simulink model "HLSDem_SelectParameter"  (R2016b)
settings: configuration reference "CodeGenConfigSet" (kept outside this file)
values from neighbouring files (symbols this model uses):
  HLSDem_facFdbkLoGrip_C = Calibration.Parameter    [init_HLSDem_SelectParameter.m]    (also in init_HLSDem_SelectParameter_SIL.m = Simulink.Parameter)
  HLSDem_facFdbkLoNoGrip_C = Calibration.Parameter    [init_HLSDem_SelectParameter.m]    (also in init_HLSDem_SelectParameter_SIL.m = Simulink.Parameter)
  HLSDem_facFdbkTrqLosHiGrip_CUR = Calibration.Parameter    [init_HLSDem_SelectParameter.m]    (also in init_HLSDem_SelectParameter_SIL.m = Simulink.Parameter)
  HLSDem_facFdbkTrqLosHiGrip_CURX = Calibration.Parameter    [init_HLSDem_SelectParameter.m]    (also in init_HLSDem_SelectParameter_SIL.m = Simulink.Parameter)
  HLSDem_facFdbkTrqLosHiNoGrip_C = Calibration.Parameter    [init_HLSDem_SelectParameter.m]    (also in init_HLSDem_SelectParameter_SIL.m = Simulink.Parameter)
  HLSDem_facFdbkTrqLosLoGrip_CUR = Calibration.Parameter    [init_HLSDem_SelectParameter.m]    (also in init_HLSDem_SelectParameter_SIL.m = Simulink.Parameter)
  HLSDem_facFdbkTrqLosLoGrip_CURX = Calibration.Parameter    [init_HLSDem_SelectParameter.m]    (also in init_HLSDem_SelectParameter_SIL.m = Simulink.Parameter)
  HLSDem_facFdbkTrqLosLoNoGrip_C = Calibration.Parameter    [init_HLSDem_SelectParameter.m]    (also in init_HLSDem_SelectParameter_SIL.m = Simulink.Parameter)
  HLSDem_facNAvrgPT1_C = Calibration.Parameter    [init_HLSDem_SelectParameter.m]    (also in init_HLSDem_SelectParameter_SIL.m = Simulink.Parameter)
  HLSDem_facTrqPT1CorFac_C = Calibration.Parameter    [init_HLSDem_SelectParameter.m]    (also in init_HLSDem_SelectParameter_SIL.m = Simulink.Parameter)
  HLSDem_GripIKiHi_CUR = Calibration.Parameter    [init_HLSDem_SelectParameter.m]    (also in init_HLSDem_SelectParameter_SIL.m = Simulink.Parameter)
  HLSDem_GripIKiHi_CURX = Calibration.Parameter    [init_HLSDem_SelectParameter.m]    (also in init_HLSDem_SelectParameter_SIL.m = Simulink.Parameter)
  HLSDem_GripIKiLo_CUR = Calibration.Parameter    [init_HLSDem_SelectParameter.m]    (also in init_HLSDem_SelectParameter_SIL.m = Simulink.Parameter)
  HLSDem_GripIKiLo_CURX = Calibration.Parameter    [init_HLSDem_SelectParameter.m]    (also in init_HLSDem_SelectParameter_SIL.m = Simulink.Parameter)
  HLSDem_GripIKiNegHi_CUR = Calibration.Parameter    [init_HLSDem_SelectParameter.m]    (also in init_HLSDem_SelectParameter_SIL.m = Simulink.Parameter)
  HLSDem_GripIKiNegHi_CURX = Calibration.Parameter    [init_HLSDem_SelectParameter.m]    (also in init_HLSDem_SelectParameter_SIL.m = Simulink.Parameter)
  HLSDem_GripIKiNegLo_CUR = Calibration.Parameter    [init_HLSDem_SelectParameter.m]    (also in init_HLSDem_SelectParameter_SIL.m = Simulink.Parameter)
  HLSDem_GripIKiNegLo_CURX = Calibration.Parameter    [init_HLSDem_SelectParameter.m]    (also in init_HLSDem_SelectParameter_SIL.m = Simulink.Parameter)
  HLSDem_GripIKiPosHi_CUR = Calibration.Parameter    [init_HLSDem_SelectParameter.m]    (also in init_HLSDem_SelectParameter_SIL.m = Simulink.Parameter)
  HLSDem_GripIKiPosHi_CURX = Calibration.Parameter    [init_HLSDem_SelectParameter.m]    (also in init_HLSDem_SelectParameter_SIL.m = Simulink.Parameter)
  HLSDem_GripIKiPosLo_CUR = Calibration.Parameter    [init_HLSDem_SelectParameter.m]    (also in init_HLSDem_SelectParameter_SIL.m = Simulink.Parameter)
  HLSDem_GripIKiPosLo_CURX = Calibration.Parameter    [init_HLSDem_SelectParameter.m]    (also in init_HLSDem_SelectParameter_SIL.m = Simulink.Parameter)
  HLSDem_GripIWinNegHi_C = Calibration.Parameter    [init_HLSDem_SelectParameter.m]    (also in init_HLSDem_SelectParameter_SIL.m = Simulink.Parameter)
  HLSDem_GripIWinNegLo_C = Calibration.Parameter    [init_HLSDem_SelectParameter.m]    (also in init_HLSDem_SelectParameter_SIL.m = Simulink.Parameter)
  HLSDem_GripIWinPosHi_C = Calibration.Parameter    [init_HLSDem_SelectParameter.m]    (also in init_HLSDem_SelectParameter_SIL.m = Simulink.Parameter)
  HLSDem_GripIWinPosLo_C = Calibration.Parameter    [init_HLSDem_SelectParameter.m]    (also in init_HLSDem_SelectParameter_SIL.m = Simulink.Parameter)
  HLSDem_GripPKpHi_CUR = Calibration.Parameter    [init_HLSDem_SelectParameter.m]    (also in init_HLSDem_SelectParameter_SIL.m = Simulink.Parameter)
  HLSDem_GripPKpHi_CURX = Calibration.Parameter    [init_HLSDem_SelectParameter.m]    (also in init_HLSDem_SelectParameter_SIL.m = Simulink.Parameter)
  HLSDem_GripPKpLo_CUR = Calibration.Parameter    [init_HLSDem_SelectParameter.m]    (also in init_HLSDem_SelectParameter_SIL.m = Simulink.Parameter)
  HLSDem_GripPKpLo_CURX = Calibration.Parameter    [init_HLSDem_SelectParameter.m]    (also in init_HLSDem_SelectParameter_SIL.m = Simulink.Parameter)
  HLSDem_GripPKpNegHi_CUR = Calibration.Parameter    [init_HLSDem_SelectParameter.m]    (also in init_HLSDem_SelectParameter_SIL.m = Simulink.Parameter)
  HLSDem_GripPKpNegHi_CURX = Calibration.Parameter    [init_HLSDem_SelectParameter.m]    (also in init_HLSDem_SelectParameter_SIL.m = Simulink.Parameter)
  HLSDem_GripPKpNegLo_CUR = Calibration.Parameter    [init_HLSDem_SelectParameter.m]    (also in init_HLSDem_SelectParameter_SIL.m = Simulink.Parameter)
  HLSDem_GripPKpNegLo_CURX = Calibration.Parameter    [init_HLSDem_SelectParameter.m]    (also in init_HLSDem_SelectParameter_SIL.m = Simulink.Parameter)
  HLSDem_GripPKpPosHi_CUR = Calibration.Parameter    [init_HLSDem_SelectParameter.m]    (also in init_HLSDem_SelectParameter_SIL.m = Simulink.Parameter)
  HLSDem_GripPKpPosHi_CURX = Calibration.Parameter    [init_HLSDem_SelectParameter.m]    (also in init_HLSDem_SelectParameter_SIL.m = Simulink.Parameter)
  HLSDem_GripPKpPosLo_CUR = Calibration.Parameter    [init_HLSDem_SelectParameter.m]    (also in init_HLSDem_SelectParameter_SIL.m = Simulink.Parameter)
  HLSDem_GripPKpPosLo_CURX = Calibration.Parameter    [init_HLSDem_SelectParameter.m]    (also in init_HLSDem_SelectParameter_SIL.m = Simulink.Parameter)
  HLSDem_GripPWinNegHi_C = Calibration.Parameter    [init_HLSDem_SelectParameter.m]    (also in init_HLSDem_SelectParameter_SIL.m = Simulink.Parameter)
  HLSDem_GripPWinNegLo_C = Calibration.Parameter    [init_HLSDem_SelectParameter.m]    (also in init_HLSDem_SelectParameter_SIL.m = Simulink.Parameter)
  HLSDem_GripPWinPosHi_C = Calibration.Parameter    [init_HLSDem_SelectParameter.m]    (also in init_HLSDem_SelectParameter_SIL.m = Simulink.Parameter)
  HLSDem_GripPWinPosLo_C = Calibration.Parameter    [init_HLSDem_SelectParameter.m]    (also in init_HLSDem_SelectParameter_SIL.m = Simulink.Parameter)
  HLSDem_InrtVehGrip_CUR = Calibration.Parameter    [init_HLSDem_SelectParameter.m]    (also in init_HLSDem_SelectParameter_SIL.m = Simulink.Parameter)
  HLSDem_InrtVehGrip_CURX = Calibration.Parameter    [init_HLSDem_SelectParameter.m]    (also in init_HLSDem_SelectParameter_SIL.m = Simulink.Parameter)
  HLSDem_InrtVehNoGrip_C = Calibration.Parameter    [init_HLSDem_SelectParameter.m]    (also in init_HLSDem_SelectParameter_SIL.m = Simulink.Parameter)
  HLSDem_KiCorFac_MAP = Calibration.Parameter    [init_HLSDem_SelectParameter.m]    (also in init_HLSDem_SelectParameter_SIL.m = Simulink.Parameter)
  HLSDem_KiCorFac_MAPX = Calibration.Parameter    [init_HLSDem_SelectParameter.m]    (also in init_HLSDem_SelectParameter_SIL.m = Simulink.Parameter)
  HLSDem_KiCorFac_MAPY = Calibration.Parameter    [init_HLSDem_SelectParameter.m]    (also in init_HLSDem_SelectParameter_SIL.m = Simulink.Parameter)
  HLSDem_KiCorTrqFac_MAP = Calibration.Parameter    [init_HLSDem_SelectParameter.m]    (also in init_HLSDem_SelectParameter_SIL.m = Simulink.Parameter)
  HLSDem_KiCorTrqFac_MAPX = Calibration.Parameter    [init_HLSDem_SelectParameter.m]    (also in init_HLSDem_SelectParameter_SIL.m = Simulink.Parameter)
  HLSDem_KiCorTrqFac_MAPY = Calibration.Parameter    [init_HLSDem_SelectParameter.m]    (also in init_HLSDem_SelectParameter_SIL.m = Simulink.Parameter)
  HLSDem_KpCorFac_MAP = Calibration.Parameter    [init_HLSDem_SelectParameter.m]    (also in init_HLSDem_SelectParameter_SIL.m = Simulink.Parameter)
  HLSDem_KpCorFac_MAPX = Calibration.Parameter    [init_HLSDem_SelectParameter.m]    (also in init_HLSDem_SelectParameter_SIL.m = Simulink.Parameter)
  HLSDem_KpCorFac_MAPY = Calibration.Parameter    [init_HLSDem_SelectParameter.m]    (also in init_HLSDem_SelectParameter_SIL.m = Simulink.Parameter)
  HLSDem_KpCorTrqFac_MAP = Calibration.Parameter    [init_HLSDem_SelectParameter.m]    (also in init_HLSDem_SelectParameter_SIL.m = Simulink.Parameter)
  HLSDem_KpCorTrqFac_MAPX = Calibration.Parameter    [init_HLSDem_SelectParameter.m]    (also in init_HLSDem_SelectParameter_SIL.m = Simulink.Parameter)
  HLSDem_KpCorTrqFac_MAPY = Calibration.Parameter    [init_HLSDem_SelectParameter.m]    (also in init_HLSDem_SelectParameter_SIL.m = Simulink.Parameter)
  HLSDem_NoGripdnAccLim_C = Calibration.Parameter    [init_HLSDem_SelectParameter.m]    (also in init_HLSDem_SelectParameter_SIL.m = Simulink.Parameter)
  HLSDem_NoGripdnDeclLim_C = Calibration.Parameter    [init_HLSDem_SelectParameter.m]    (also in init_HLSDem_SelectParameter_SIL.m = Simulink.Parameter)
  HLSDem_NoGripdnDeclLimBrk_C = Calibration.Parameter    [init_HLSDem_SelectParameter.m]    (also in init_HLSDem_SelectParameter_SIL.m = Simulink.Parameter)
  HLSDem_NoGripIKiHi_C = Calibration.Parameter    [init_HLSDem_SelectParameter.m]    (also in init_HLSDem_SelectParameter_SIL.m = Simulink.Parameter)
  HLSDem_NoGripIKiLo_C = Calibration.Parameter    [init_HLSDem_SelectParameter.m]    (also in init_HLSDem_SelectParameter_SIL.m = Simulink.Parameter)
  HLSDem_NoGripIKiNegHi_C = Calibration.Parameter    [init_HLSDem_SelectParameter.m]    (also in init_HLSDem_SelectParameter_SIL.m = Simulink.Parameter)
  HLSDem_NoGripIKiNegLo_C = Calibration.Parameter    [init_HLSDem_SelectParameter.m]    (also in init_HLSDem_SelectParameter_SIL.m = Simulink.Parameter)
  HLSDem_NoGripIKiPosHi_C = Calibration.Parameter    [init_HLSDem_SelectParameter.m]    (also in init_HLSDem_SelectParameter_SIL.m = Simulink.Parameter)
  HLSDem_NoGripIKiPosLo_C = Calibration.Parameter    [init_HLSDem_SelectParameter.m]    (also in init_HLSDem_SelectParameter_SIL.m = Simulink.Parameter)
  HLSDem_NoGripIWinNegHi_C = Calibration.Parameter    [init_HLSDem_SelectParameter.m]    (also in init_HLSDem_SelectParameter_SIL.m = Simulink.Parameter)
  HLSDem_NoGripIWinNegLo_C = Calibration.Parameter    [init_HLSDem_SelectParameter.m]    (also in init_HLSDem_SelectParameter_SIL.m = Simulink.Parameter)
  HLSDem_NoGripIWinPosHi_C = Calibration.Parameter    [init_HLSDem_SelectParameter.m]    (also in init_HLSDem_SelectParameter_SIL.m = Simulink.Parameter)
  HLSDem_NoGripIWinPosLo_C = Calibration.Parameter    [init_HLSDem_SelectParameter.m]    (also in init_HLSDem_SelectParameter_SIL.m = Simulink.Parameter)
  HLSDem_NoGripPKpHi_C = Calibration.Parameter    [init_HLSDem_SelectParameter.m]    (also in init_HLSDem_SelectParameter_SIL.m = Simulink.Parameter)
  HLSDem_NoGripPKpLo_C = Calibration.Parameter    [init_HLSDem_SelectParameter.m]    (also in init_HLSDem_SelectParameter_SIL.m = Simulink.Parameter)
  HLSDem_NoGripPKpNegHi_C = Calibration.Parameter    [init_HLSDem_SelectParameter.m]    (also in init_HLSDem_SelectParameter_SIL.m = Simulink.Parameter)
  HLSDem_NoGripPKpNegLo_C = Calibration.Parameter    [init_HLSDem_SelectParameter.m]    (also in init_HLSDem_SelectParameter_SIL.m = Simulink.Parameter)
  HLSDem_NoGripPKpPosHi_C = Calibration.Parameter    [init_HLSDem_SelectParameter.m]    (also in init_HLSDem_SelectParameter_SIL.m = Simulink.Parameter)
  HLSDem_NoGripPKpPosLo_C = Calibration.Parameter    [init_HLSDem_SelectParameter.m]    (also in init_HLSDem_SelectParameter_SIL.m = Simulink.Parameter)
  HLSDem_NoGripPWinNegHi_C = Calibration.Parameter    [init_HLSDem_SelectParameter.m]    (also in init_HLSDem_SelectParameter_SIL.m = Simulink.Parameter)
  HLSDem_NoGripPWinNegLo_C = Calibration.Parameter    [init_HLSDem_SelectParameter.m]    (also in init_HLSDem_SelectParameter_SIL.m = Simulink.Parameter)
  HLSDem_NoGripPWinPosHi_C = Calibration.Parameter    [init_HLSDem_SelectParameter.m]    (also in init_HLSDem_SelectParameter_SIL.m = Simulink.Parameter)
  HLSDem_NoGripPWinPosLo_C = Calibration.Parameter    [init_HLSDem_SelectParameter.m]    (also in init_HLSDem_SelectParameter_SIL.m = Simulink.Parameter)
  HLSDem_rNoGripThres_C = Calibration.Parameter    [init_HLSDem_SelectParameter.m]    (also in init_HLSDem_SelectParameter_SIL.m = Simulink.Parameter)
  HLSDem_stBrkTrq_C = Calibration.Parameter    [init_HLSDem_SelectParameter.m]    (also in init_HLSDem_SelectParameter_SIL.m = Simulink.Parameter)
  HLSDem_swtTempSelParAdap_C = Calibration.Parameter    [init_HLSDem_SelectParameter.m]    (also in init_HLSDem_SelectParameter_SIL.m = Simulink.Parameter)
  HLSDem_swtTrqSelCorFac_C = Calibration.Parameter    [init_HLSDem_SelectParameter.m]    (also in init_HLSDem_SelectParameter_SIL.m = Simulink.Parameter)
  HLSDem_tiFltTrqLosGrip_CUR = Calibration.Parameter    [init_HLSDem_SelectParameter.m]    (also in init_HLSDem_SelectParameter_SIL.m = Simulink.Parameter)
  HLSDem_tiFltTrqLosGrip_CURX = Calibration.Parameter    [init_HLSDem_SelectParameter.m]    (also in init_HLSDem_SelectParameter_SIL.m = Simulink.Parameter)
  HLSDem_tiFltTrqLosNoGrip_C = Calibration.Parameter    [init_HLSDem_SelectParameter.m]    (also in init_HLSDem_SelectParameter_SIL.m = Simulink.Parameter)
libraries: CXLib x2
(part 1 of 2)
settings Model: Creator=Administrator  LastModifiedBy=xuxingpei
settings ConfigSetRef: SourceLocation=Base Workspace

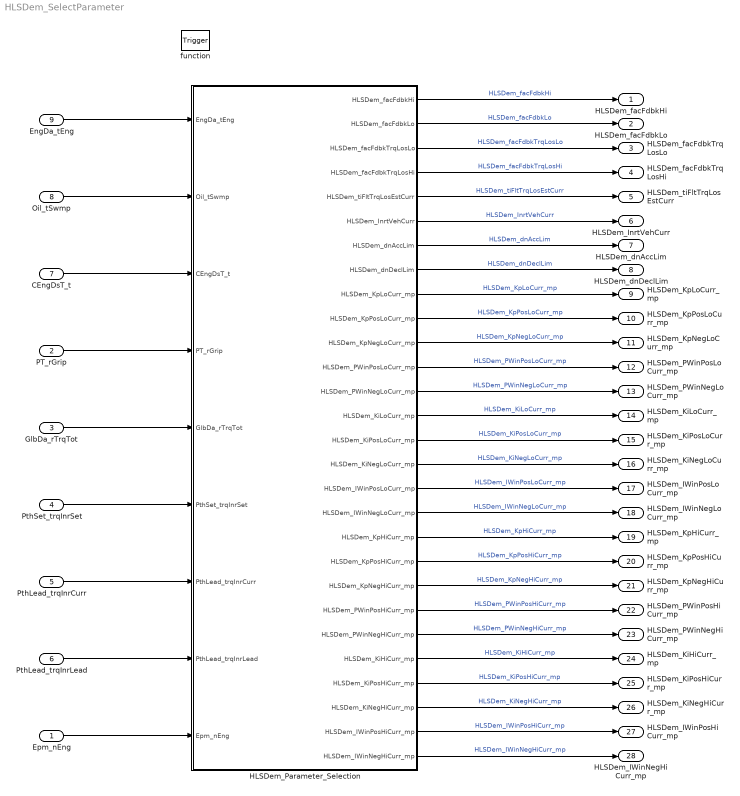
== system HLSDem_SelectParameter ==
  Epm_nEng : Inport  Tag=rpm  Description=Engine speed  OutMin=0  OutMax=6000  OutDataTypeStr=EngSpeed_rpm
  PT_rGrip : Inport  Description=Analogue value for the grip states  Port=2  OutMin=-300  OutMax=300  OutDataTypeStr=Prc_Fact100
  GlbDa_rTrqTot : Inport  Description=total ratio of the power train inclusive the differential and the converter torque ratio  Port=3  OutMin=-327  OutMax=327  OutDataTypeStr=TransRatio
  PthSet_trqInrSet : Inport  Tag=Nm  Description=Inner torque set value after monitoring limitation  Port=4  OutMin=-3000  OutMax=3276.7  OutDataTypeStr=Trq_Nm
  PthLead_trqInrCurr : Inport  Tag=Nm  Description=Actual percent engine torque  Port=5  OutMin=-3000  OutMax=3000  OutDataTypeStr=Trq_Nm
  PthLead_trqInrLead : Inport  Tag=Nm  Description=Inner torque lead value  Port=6  OutMin=-3000  OutMax=3000  OutDataTypeStr=Trq_Nm
  CEngDsT_t : Inport  Tag=deg  Description=engine coolant temperature after filter  Port=7  OutMin=-200  OutMax=200  OutDataTypeStr=Temp_deg
  Oil_tSwmp : Inport  Tag=deg  Description=Oil temperature in oil sump  Port=8  OutMin=-50  OutMax=200  OutDataTypeStr=Temp_deg
  EngDa_tEng : Inport  Tag=deg  Description=Engine temperature  Port=9  OutMin=-1000  OutMax=1000  OutDataTypeStr=Temp_deg
  function : TriggerPort  TriggerType=function-call  VariantControl=Variant
  HLSDem_Parameter_Selection : Subsystem
  HLSDem_facFdbkHi : Outport  Tag=rpm/Nm  Description=Feedback factor for the upper setpoint  OutMin=-20  OutMax=20  OutDataTypeStr=FdbkNm2rpm_rpm_Nm
  HLSDem_facFdbkLo : Outport  Tag=rpm/Nm  Description=Feedback factor for the lower setpoint  Port=2  OutMin=-20  OutMax=20  OutDataTypeStr=FdbkNm2rpm_rpm_Nm
  HLSDem_facFdbkTrqLosLo : Outport  Tag=rpm/Nm  Description=Inner feedback factor for the lower setpoint  Port=3  OutMin=-20  OutMax=20  OutDataTypeStr=FdbkNm2rpm_rpm_Nm
  HLSDem_facFdbkTrqLosHi : Outport  Tag=rpm/Nm  Description=Inner feedback factor for the upper setpoint  Port=4  OutMin=-20  OutMax=20  OutDataTypeStr=FdbkNm2rpm_rpm_Nm
  HLSDem_tiFltTrqLosEstCurr : Outport  Description=Time constant (PT1filter) for EISGov torque loss estimation  Port=5  OutMin=0  OutMax=99.998  OutDataTypeStr=PT_fac
  HLSDem_InrtVehCurr : Outport  Tag=Nm/(rpm/s)  Description=Mass Inertia for EISGov torque loss estimation  Port=6  OutMin=-50  OutMax=50  OutDataTypeStr=HLSDem_Inrt
  HLSDem_dnAccLim : Outport  Tag=rpm/s  Description=Maximum permissible acceleration (Engine speed)  Port=7  OutMin=-12000  OutMax=12000  OutDataTypeStr=EngSpeed_rpm_s
  HLSDem_dnDeclLim : Outport  Tag=rpm/s  Description=Maximum permissible deceleration (Engine speed)  Port=8  OutMin=-12000  OutMax=12000  OutDataTypeStr=EngSpeed_rpm_s
  HLSDem_KpLoCurr_mp : Outport  Tag=Nm/rpm  Description=Current gain of the P-element of lower path  Port=9  OutMin=-10000  OutMax=10000  OutDataTypeStr=HLSDem_Kp
  HLSDem_KpPosLoCurr_mp : Outport  Tag=Nm/rpm  Description=Current positive large signal gain of the P-element of lower path  Port=10  OutMin=-10000  OutMax=10000  OutDataTypeStr=HLSDem_Kp
  HLSDem_KpNegLoCurr_mp : Outport  Tag=Nm/rpm  Description=Current negative large signal gain of the P-element of lower path  Port=11  OutMin=-10000  OutMax=10000  OutDataTypeStr=HLSDem_Kp
  HLSDem_PWinPosLoCurr_mp : Outport  Tag=rpm  Description=Current positive small-signal window P-component of the lower path  Port=12  OutMin=-6000  OutMax=6000  OutDataTypeStr=EngSpeed_rpm
  HLSDem_PWinNegLoCurr_mp : Outport  Tag=rpm  Description=Current negative small-signal window P-component of the lower path  Port=13  OutMin=-6000  OutMax=6000  OutDataTypeStr=EngSpeed_rpm
  HLSDem_KiLoCurr_mp : Outport  Tag=Nm/(rpm*s)  Description=Current gain of the I-element of lower path  Port=14  OutMin=-18000  OutMax=18000  OutDataTypeStr=HLSDem_Ki
  HLSDem_KiPosLoCurr_mp : Outport  Tag=Nm/(rpm*s)  Description=Current positive large signal gain of the I-element of lower path  Port=15  OutMin=-18000  OutMax=18000  OutDataTypeStr=HLSDem_Ki
  HLSDem_KiNegLoCurr_mp : Outport  Tag=Nm/(rpm*s)  Description=Current negative large signal gain of the I-element of lower path  Port=16  OutMin=-18000  OutMax=18000  OutDataTypeStr=HLSDem_Ki
  HLSDem_IWinPosLoCurr_mp : Outport  Tag=rpm  Description=Current positive small-signal window I-component of the lower path  Port=17  OutMin=-6000  OutMax=6000  OutDataTypeStr=EngSpeed_rpm
  HLSDem_IWinNegLoCurr_mp : Outport  Tag=rpm  Description=Current negative small-signal window I-component of the lower path  Port=18  OutMin=-6000  OutMax=6000  OutDataTypeStr=EngSpeed_rpm
  HLSDem_KpHiCurr_mp : Outport  Tag=Nm/rpm  Description=Current gain of the P-element of upper path  Port=19  OutMin=-10000  OutMax=10000  OutDataTypeStr=HLSDem_Kp
  HLSDem_KpPosHiCurr_mp : Outport  Tag=Nm/rpm  Description=Current positive large signal gain of the P-element of upper path  Port=20  OutMin=-10000  OutMax=10000  OutDataTypeStr=HLSDem_Kp
  HLSDem_KpNegHiCurr_mp : Outport  Tag=Nm/rpm  Description=Current negative large signal gain of the P-element of upper path  Port=21  OutMin=-10000  OutMax=10000  OutDataTypeStr=HLSDem_Kp
  HLSDem_PWinPosHiCurr_mp : Outport  Tag=rpm  Description=Current positive small-signal window P-component of the upper path  Port=22  OutMin=-6000  OutMax=6000  OutDataTypeStr=EngSpeed_rpm
  HLSDem_PWinNegHiCurr_mp : Outport  Tag=rpm  Description=Current negative small-signal window P-component of the upper path  Port=23  OutMin=-6000  OutMax=6000  OutDataTypeStr=EngSpeed_rpm
  HLSDem_KiHiCurr_mp : Outport  Tag=Nm/(rpm*s)  Description=Current small signal gain for the I component upper PI - path  Port=24  OutMin=-18000  OutMax=18000  OutDataTypeStr=HLSDem_Ki
  HLSDem_KiPosHiCurr_mp : Outport  Tag=Nm/(rpm*s)  Description=Current positive large signal gain for the I component upper PI-path  Port=25  OutMin=-18000  OutMax=18000  OutDataTypeStr=HLSDem_Ki
  HLSDem_KiNegHiCurr_mp : Outport  Tag=Nm/(rpm*s)  Description=Current negative large signal gain for the I component upper PI - path  Port=26  OutMin=-18000  OutMax=18000  OutDataTypeStr=HLSDem_Ki
  HLSDem_IWinPosHiCurr_mp : Outport  Tag=rpm  Description=Current positive small-signal window I-component of the upper path  Port=27  OutMin=-6000  OutMax=6000  OutDataTypeStr=EngSpeed_rpm
  HLSDem_IWinNegHiCurr_mp : Outport  Tag=rpm  Description=Current negative small-signal window I-component of the upper path  Port=28  OutMin=-6000  OutMax=6000  OutDataTypeStr=EngSpeed_rpm
  wires:
  PT_rGrip/1 -> HLSDem_Parameter_Selection/4(PT_rGrip)
  PthSet_trqInrSet/1 -> HLSDem_Parameter_Selection/6(PthSet_trqInrSet)
  Epm_nEng/1 -> HLSDem_Parameter_Selection/9(Epm_nEng)
  PthLead_trqInrCurr/1 -> HLSDem_Parameter_Selection/7(PthLead_trqInrCurr)
  PthLead_trqInrLead/1 -> HLSDem_Parameter_Selection/8(PthLead_trqInrLead)
  GlbDa_rTrqTot/1 -> HLSDem_Parameter_Selection/5(GlbDa_rTrqTot)
  HLSDem_Parameter_Selection/1(HLSDem_facFdbkHi) -> HLSDem_facFdbkHi/1  "HLSDem_facFdbkHi"
  HLSDem_Parameter_Selection/2(HLSDem_facFdbkLo) -> HLSDem_facFdbkLo/1  "HLSDem_facFdbkLo"
  HLSDem_Parameter_Selection/3(HLSDem_facFdbkTrqLosLo) -> HLSDem_facFdbkTrqLosLo/1  "HLSDem_facFdbkTrqLosLo"
  HLSDem_Parameter_Selection/4(HLSDem_facFdbkTrqLosHi) -> HLSDem_facFdbkTrqLosHi/1  "HLSDem_facFdbkTrqLosHi"
  HLSDem_Parameter_Selection/5(HLSDem_tiFltTrqLosEstCurr) -> HLSDem_tiFltTrqLosEstCurr/1  "HLSDem_tiFltTrqLosEstCurr"
  HLSDem_Parameter_Selection/6(HLSDem_InrtVehCurr) -> HLSDem_InrtVehCurr/1  "HLSDem_InrtVehCurr"
  HLSDem_Parameter_Selection/7(HLSDem_dnAccLim) -> HLSDem_dnAccLim/1  "HLSDem_dnAccLim"
  HLSDem_Parameter_Selection/8(HLSDem_dnDeclLim) -> HLSDem_dnDeclLim/1  "HLSDem_dnDeclLim"
  HLSDem_Parameter_Selection/9(HLSDem_KpLoCurr_mp) -> HLSDem_KpLoCurr_mp/1  "HLSDem_KpLoCurr_mp"
  HLSDem_Parameter_Selection/10(HLSDem_KpPosLoCurr_mp) -> HLSDem_KpPosLoCurr_mp/1  "HLSDem_KpPosLoCurr_mp"
  HLSDem_Parameter_Selection/11(HLSDem_KpNegLoCurr_mp) -> HLSDem_KpNegLoCurr_mp/1  "HLSDem_KpNegLoCurr_mp"
  HLSDem_Parameter_Selection/12(HLSDem_PWinPosLoCurr_mp) -> HLSDem_PWinPosLoCurr_mp/1  "HLSDem_PWinPosLoCurr_mp"
  HLSDem_Parameter_Selection/13(HLSDem_PWinNegLoCurr_mp) -> HLSDem_PWinNegLoCurr_mp/1  "HLSDem_PWinNegLoCurr_mp"
  HLSDem_Parameter_Selection/14(HLSDem_KiLoCurr_mp) -> HLSDem_KiLoCurr_mp/1  "HLSDem_KiLoCurr_mp"
  HLSDem_Parameter_Selection/15(HLSDem_KiPosLoCurr_mp) -> HLSDem_KiPosLoCurr_mp/1  "HLSDem_KiPosLoCurr_mp"
  HLSDem_Parameter_Selection/16(HLSDem_KiNegLoCurr_mp) -> HLSDem_KiNegLoCurr_mp/1  "HLSDem_KiNegLoCurr_mp"
  HLSDem_Parameter_Selection/17(HLSDem_IWinPosLoCurr_mp) -> HLSDem_IWinPosLoCurr_mp/1  "HLSDem_IWinPosLoCurr_mp"
  HLSDem_Parameter_Selection/18(HLSDem_IWinNegLoCurr_mp) -> HLSDem_IWinNegLoCurr_mp/1  "HLSDem_IWinNegLoCurr_mp"
  HLSDem_Parameter_Selection/19(HLSDem_KpHiCurr_mp) -> HLSDem_KpHiCurr_mp/1  "HLSDem_KpHiCurr_mp"
  HLSDem_Parameter_Selection/20(HLSDem_KpPosHiCurr_mp) -> HLSDem_KpPosHiCurr_mp/1  "HLSDem_KpPosHiCurr_mp"
  HLSDem_Parameter_Selection/21(HLSDem_KpNegHiCurr_mp) -> HLSDem_KpNegHiCurr_mp/1  "HLSDem_KpNegHiCurr_mp"
  HLSDem_Parameter_Selection/22(HLSDem_PWinPosHiCurr_mp) -> HLSDem_PWinPosHiCurr_mp/1  "HLSDem_PWinPosHiCurr_mp"
  HLSDem_Parameter_Selection/23(HLSDem_PWinNegHiCurr_mp) -> HLSDem_PWinNegHiCurr_mp/1  "HLSDem_PWinNegHiCurr_mp"
  HLSDem_Parameter_Selection/24(HLSDem_KiHiCurr_mp) -> HLSDem_KiHiCurr_mp/1  "HLSDem_KiHiCurr_mp"
  HLSDem_Parameter_Selection/25(HLSDem_KiPosHiCurr_mp) -> HLSDem_KiPosHiCurr_mp/1  "HLSDem_KiPosHiCurr_mp"
  HLSDem_Parameter_Selection/26(HLSDem_KiNegHiCurr_mp) -> HLSDem_KiNegHiCurr_mp/1  "HLSDem_KiNegHiCurr_mp"
  HLSDem_Parameter_Selection/27(HLSDem_IWinPosHiCurr_mp) -> HLSDem_IWinPosHiCurr_mp/1  "HLSDem_IWinPosHiCurr_mp"
  HLSDem_Parameter_Selection/28(HLSDem_IWinNegHiCurr_mp) -> HLSDem_IWinNegHiCurr_mp/1  "HLSDem_IWinNegHiCurr_mp"
  CEngDsT_t/1 -> HLSDem_Parameter_Selection/3(CEngDsT_t)
  Oil_tSwmp/1 -> HLSDem_Parameter_Selection/2(Oil_tSwmp)
  EngDa_tEng/1 -> HLSDem_Parameter_Selection/1(EngDa_tEng)

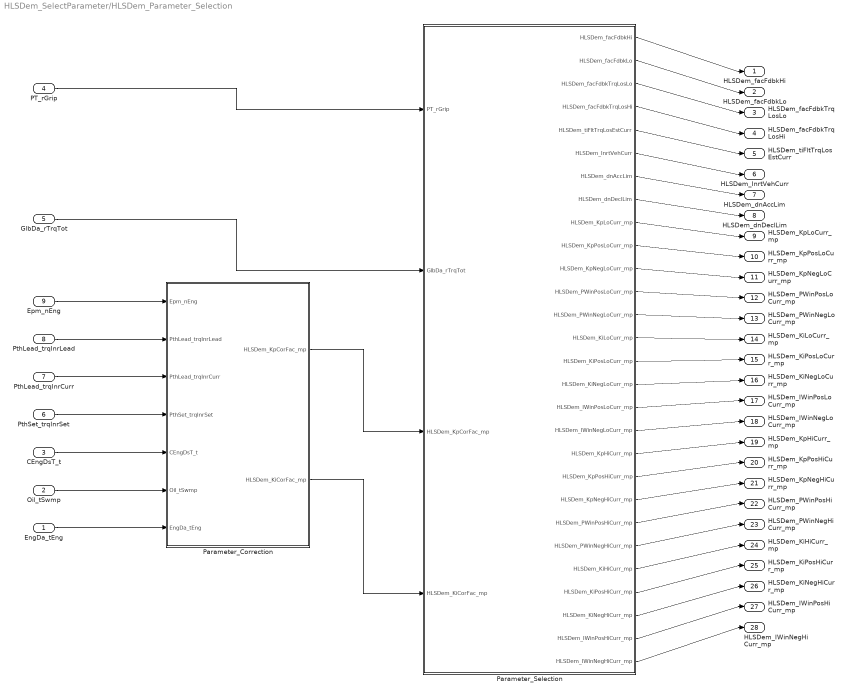
== system HLSDem_SelectParameter/HLSDem_Parameter_Selection ==
  EngDa_tEng : Inport  Tag=deg  Description=Engine temperature  OutMin=-1000  OutMax=1000  OutDataTypeStr=Temp_deg
  Oil_tSwmp : Inport  Tag=deg  Description=Oil temperature in oil sump  Port=2  OutMin=-50  OutMax=200  OutDataTypeStr=Temp_deg
  CEngDsT_t : Inport  Tag=deg  Description=engine coolant temperature after filter  Port=3  OutMin=-200  OutMax=200  OutDataTypeStr=Temp_deg
  PT_rGrip : Inport  Port=4
  GlbDa_rTrqTot : Inport  Port=5
  PthSet_trqInrSet : Inport  Port=6
  PthLead_trqInrCurr : Inport  Port=7
  PthLead_trqInrLead : Inport  Port=8
  Epm_nEng : Inport  Port=9
  Parameter_Correction : Subsystem
  Parameter_Selection : Subsystem
  HLSDem_facFdbkHi : Outport
  HLSDem_facFdbkLo : Outport  Port=2
  HLSDem_facFdbkTrqLosLo : Outport  Port=3
  HLSDem_facFdbkTrqLosHi : Outport  Port=4
  HLSDem_tiFltTrqLosEstCurr : Outport  Port=5
  HLSDem_InrtVehCurr : Outport  Port=6
  HLSDem_dnAccLim : Outport  Port=7
  HLSDem_dnDeclLim : Outport  Port=8
  HLSDem_KpLoCurr_mp : Outport  Port=9
  HLSDem_KpPosLoCurr_mp : Outport  Port=10
  HLSDem_KpNegLoCurr_mp : Outport  Port=11
  HLSDem_PWinPosLoCurr_mp : Outport  Port=12
  HLSDem_PWinNegLoCurr_mp : Outport  Port=13
  HLSDem_KiLoCurr_mp : Outport  Port=14
  HLSDem_KiPosLoCurr_mp : Outport  Port=15
  HLSDem_KiNegLoCurr_mp : Outport  Port=16
  HLSDem_IWinPosLoCurr_mp : Outport  Port=17
  HLSDem_IWinNegLoCurr_mp : Outport  Port=18
  HLSDem_KpHiCurr_mp : Outport  Port=19
  HLSDem_KpPosHiCurr_mp : Outport  Port=20
  HLSDem_KpNegHiCurr_mp : Outport  Port=21
  HLSDem_PWinPosHiCurr_mp : Outport  Port=22
  HLSDem_PWinNegHiCurr_mp : Outport  Port=23
  HLSDem_KiHiCurr_mp : Outport  Port=24
  HLSDem_KiPosHiCurr_mp : Outport  Port=25
  HLSDem_KiNegHiCurr_mp : Outport  Port=26
  HLSDem_IWinPosHiCurr_mp : Outport  Port=27
  HLSDem_IWinNegHiCurr_mp : Outport  Port=28
  wires:
  Parameter_Correction/2(HLSDem_KiCorFac_mp) -> Parameter_Selection/4(HLSDem_KiCorFac_mp)
  Epm_nEng/1 -> Parameter_Correction/1(Epm_nEng)
  PT_rGrip/1 -> Parameter_Selection/1(PT_rGrip)
  GlbDa_rTrqTot/1 -> Parameter_Selection/2(GlbDa_rTrqTot)
  PthLead_trqInrLead/1 -> Parameter_Correction/2(PthLead_trqInrLead)
  PthSet_trqInrSet/1 -> Parameter_Correction/4(PthSet_trqInrSet)
  PthLead_trqInrCurr/1 -> Parameter_Correction/3(PthLead_trqInrCurr)
  Parameter_Correction/1(HLSDem_KpCorFac_mp) -> Parameter_Selection/3(HLSDem_KpCorFac_mp)
  Parameter_Selection/1(HLSDem_facFdbkHi) -> HLSDem_facFdbkHi/1
  Parameter_Selection/2(HLSDem_facFdbkLo) -> HLSDem_facFdbkLo/1
  Parameter_Selection/3(HLSDem_facFdbkTrqLosLo) -> HLSDem_facFdbkTrqLosLo/1
  Parameter_Selection/4(HLSDem_facFdbkTrqLosHi) -> HLSDem_facFdbkTrqLosHi/1
  Parameter_Selection/5(HLSDem_tiFltTrqLosEstCurr) -> HLSDem_tiFltTrqLosEstCurr/1
  Parameter_Selection/6(HLSDem_InrtVehCurr) -> HLSDem_InrtVehCurr/1
  Parameter_Selection/7(HLSDem_dnAccLim) -> HLSDem_dnAccLim/1
  Parameter_Selection/8(HLSDem_dnDeclLim) -> HLSDem_dnDeclLim/1
  Parameter_Selection/9(HLSDem_KpLoCurr_mp) -> HLSDem_KpLoCurr_mp/1
  Parameter_Selection/10(HLSDem_KpPosLoCurr_mp) -> HLSDem_KpPosLoCurr_mp/1
  Parameter_Selection/11(HLSDem_KpNegLoCurr_mp) -> HLSDem_KpNegLoCurr_mp/1
  Parameter_Selection/12(HLSDem_PWinPosLoCurr_mp) -> HLSDem_PWinPosLoCurr_mp/1
  Parameter_Selection/13(HLSDem_PWinNegLoCurr_mp) -> HLSDem_PWinNegLoCurr_mp/1
  Parameter_Selection/14(HLSDem_KiLoCurr_mp) -> HLSDem_KiLoCurr_mp/1
  Parameter_Selection/15(HLSDem_KiPosLoCurr_mp) -> HLSDem_KiPosLoCurr_mp/1
  Parameter_Selection/16(HLSDem_KiNegLoCurr_mp) -> HLSDem_KiNegLoCurr_mp/1
  Parameter_Selection/17(HLSDem_IWinPosLoCurr_mp) -> HLSDem_IWinPosLoCurr_mp/1
  Parameter_Selection/18(HLSDem_IWinNegLoCurr_mp) -> HLSDem_IWinNegLoCurr_mp/1
  Parameter_Selection/19(HLSDem_KpHiCurr_mp) -> HLSDem_KpHiCurr_mp/1
  Parameter_Selection/20(HLSDem_KpPosHiCurr_mp) -> HLSDem_KpPosHiCurr_mp/1
  Parameter_Selection/21(HLSDem_KpNegHiCurr_mp) -> HLSDem_KpNegHiCurr_mp/1
  Parameter_Selection/22(HLSDem_PWinPosHiCurr_mp) -> HLSDem_PWinPosHiCurr_mp/1
  Parameter_Selection/23(HLSDem_PWinNegHiCurr_mp) -> HLSDem_PWinNegHiCurr_mp/1
  Parameter_Selection/24(HLSDem_KiHiCurr_mp) -> HLSDem_KiHiCurr_mp/1
  Parameter_Selection/25(HLSDem_KiPosHiCurr_mp) -> HLSDem_KiPosHiCurr_mp/1
  Parameter_Selection/26(HLSDem_KiNegHiCurr_mp) -> HLSDem_KiNegHiCurr_mp/1
  Parameter_Selection/27(HLSDem_IWinPosHiCurr_mp) -> HLSDem_IWinPosHiCurr_mp/1
  Parameter_Selection/28(HLSDem_IWinNegHiCurr_mp) -> HLSDem_IWinNegHiCurr_mp/1
  Oil_tSwmp/1 -> Parameter_Correction/6(Oil_tSwmp)
  EngDa_tEng/1 -> Parameter_Correction/7(EngDa_tEng)
  CEngDsT_t/1 -> Parameter_Correction/5(CEngDsT_t)

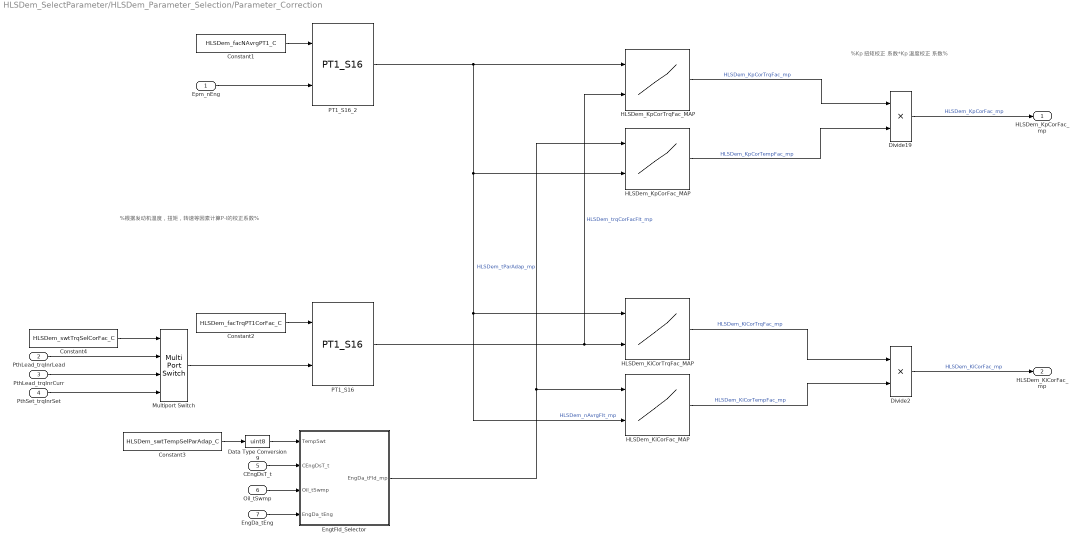
== system HLSDem_SelectParameter/HLSDem_Parameter_Selection/Parameter_Correction ==
  note: %Kp 扭矩校正 系数*Kp 温度校正 系数%
  note: %根据发动机温度，扭矩，转速等因素计算P-I的校正系数%
  Epm_nEng : Inport
  PthLead_trqInrLead : Inport  Port=2
  PthLead_trqInrCurr : Inport  Port=3
  PthSet_trqInrSet : Inport  Port=4
  CEngDsT_t : Inport  Tag=deg  Description=engine coolant temperature after filter  Port=5  OutMin=-200  OutMax=200  OutDataTypeStr=Temp_deg
  Oil_tSwmp : Inport  Tag=deg  Description=Oil temperature in oil sump  Port=6  OutMin=-50  OutMax=200  OutDataTypeStr=Temp_deg
  EngDa_tEng : Inport  Tag=deg  Description=Engine temperature  Port=7  OutMin=-1000  OutMax=1000  OutDataTypeStr=Temp_deg
  Constant1 : Constant  Value=HLSDem_facNAvrgPT1_C
  Constant2 : Constant  Value=HLSDem_facTrqPT1CorFac_C
  Constant3 : Constant  Value=HLSDem_swtTempSelParAdap_C
  Constant4 : Constant  Value=HLSDem_swtTrqSelCorFac_C
  Data Type Conversion9 : DataTypeConversion  OutDataTypeStr=uint8
  Divide19 : Product  Inputs=**  OutDataTypeStr=Factor  SaturateOnIntegerOverflow=on
  Divide2 : Product  Inputs=**  OutDataTypeStr=Factor  SaturateOnIntegerOverflow=on
  EngtFld_Selector : Subsystem
  HLSDem_KiCorFac_MAP : Lookup_n-D  BreakpointsForDimension1=HLSDem_KiCorFac_MAPY  BreakpointsForDimension2=HLSDem_KiCorFac_MAPX  Table=HLSDem_KiCorFac_MAP  ExtrapMethod=Clip  InternalRulePriority=Speed  OutDataTypeStr=Inherit: Inherit via back propagation  RndMeth=Simplest  SaturateOnIntegerOverflow=on
  HLSDem_KiCorTrqFac_MAP : Lookup_n-D  BreakpointsForDimension1=HLSDem_KiCorTrqFac_MAPY  BreakpointsForDimension2=HLSDem_KiCorTrqFac_MAPX  Table=HLSDem_KiCorTrqFac_MAP  ExtrapMethod=Clip  InternalRulePriority=Speed  OutDataTypeStr=Inherit: Inherit via back propagation  RndMeth=Simplest  SaturateOnIntegerOverflow=on
  HLSDem_KpCorFac_MAP : Lookup_n-D  BreakpointsForDimension1=HLSDem_KpCorFac_MAPY  BreakpointsForDimension2=HLSDem_KpCorFac_MAPX  Table=HLSDem_KpCorFac_MAP  ExtrapMethod=Clip  InternalRulePriority=Speed  OutDataTypeStr=Inherit: Inherit via back propagation  RndMeth=Simplest  SaturateOnIntegerOverflow=on
  HLSDem_KpCorTrqFac_MAP : Lookup_n-D  BreakpointsForDimension1=HLSDem_KpCorTrqFac_MAPY  BreakpointsForDimension2=HLSDem_KpCorTrqFac_MAPX  Table=HLSDem_KpCorTrqFac_MAP  ExtrapMethod=Clip  InternalRulePriority=Speed  OutDataTypeStr=Inherit: Inherit via back propagation  RndMeth=Simplest  SaturateOnIntegerOverflow=on
  Multiport Switch : MultiPortSwitch  DataPortOrder=Specify indices  DataPortIndices={2,1,0}
  PT1_S16 : CXLib/PT1_S16
  PT1_S16_2 : CXLib/PT1_S16
  HLSDem_KpCorFac_mp : Outport
  HLSDem_KiCorFac_mp : Outport  Port=2
  wires:
  PT1_S16/1 -> HLSDem_KiCorTrqFac_MAP/2, HLSDem_KpCorTrqFac_MAP/2  "HLSDem_trqCorFacFlt_mp"
  PthLead_trqInrCurr/1 -> Multiport Switch/3
  Epm_nEng/1 -> PT1_S16_2/2
  HLSDem_KiCorTrqFac_MAP/1 -> Divide2/1  "HLSDem_KiCorTrqFac_mp"
  Multiport Switch/1 -> PT1_S16/2
  PthSet_trqInrSet/1 -> Multiport Switch/4
  Constant4/1 -> Multiport Switch/1
  Constant1/1 -> PT1_S16_2/1
  HLSDem_KpCorFac_MAP/1 -> Divide19/2  "HLSDem_KpCorTempFac_mp"
  HLSDem_KiCorFac_MAP/1 -> Divide2/2  "HLSDem_KiCorTempFac_mp"
  Divide19/1 -> HLSDem_KpCorFac_mp/1  "HLSDem_KpCorFac_mp"
  Constant3/1 -> Data Type Conversion9/1
  HLSDem_KpCorTrqFac_MAP/1 -> Divide19/1  "HLSDem_KpCorTrqFac_mp"
  EngtFld_Selector/1(EngDa_tFld_mp) -> HLSDem_KiCorFac_MAP/1, HLSDem_KpCorFac_MAP/1  "HLSDem_tParAdap_mp"
  PT1_S16_2/1 -> HLSDem_KiCorFac_MAP/2, HLSDem_KiCorTrqFac_MAP/1, HLSDem_KpCorFac_MAP/2, HLSDem_KpCorTrqFac_MAP/1  "HLSDem_nAvrgFlt_mp"
  PthLead_trqInrLead/1 -> Multiport Switch/2
  Constant2/1 -> PT1_S16/1
  Divide2/1 -> HLSDem_KiCorFac_mp/1  "HLSDem_KiCorFac_mp"
  Data Type Conversion9/1 -> EngtFld_Selector/1(TempSwt)
  CEngDsT_t/1 -> EngtFld_Selector/2(CEngDsT_t)
  Oil_tSwmp/1 -> EngtFld_Selector/3(Oil_tSwmp)
  EngDa_tEng/1 -> EngtFld_Selector/4(EngDa_tEng)

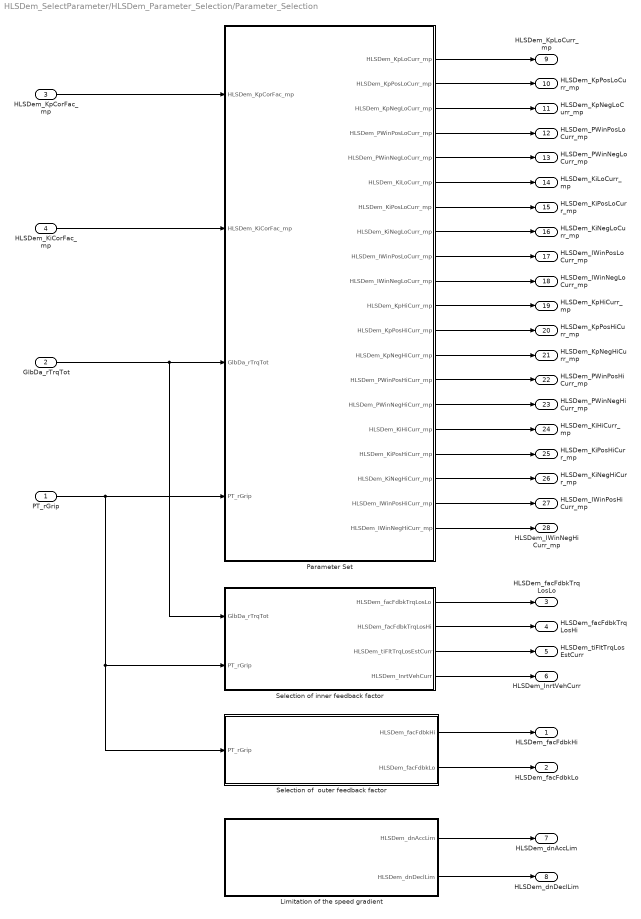
== system HLSDem_SelectParameter/HLSDem_Parameter_Selection/Parameter_Selection ==
  PT_rGrip : Inport
  GlbDa_rTrqTot : Inport  Port=2
  HLSDem_KpCorFac_mp : Inport  Port=3
  HLSDem_KiCorFac_mp : Inport  Port=4
  Limitation of the speed gradient : Subsystem
  Parameter Set : Subsystem
  Selection of  outer feedback factor : Subsystem
  Selection of inner feedback factor : Subsystem
  HLSDem_facFdbkHi : Outport
  HLSDem_facFdbkLo : Outport  Port=2
  HLSDem_facFdbkTrqLosLo : Outport  Port=3
  HLSDem_facFdbkTrqLosHi : Outport  Port=4
  HLSDem_tiFltTrqLosEstCurr : Outport  Port=5
  HLSDem_InrtVehCurr : Outport  Port=6
  HLSDem_dnAccLim : Outport  Port=7
  HLSDem_dnDeclLim : Outport  Port=8
  HLSDem_KpLoCurr_mp : Outport  Port=9
  HLSDem_KpPosLoCurr_mp : Outport  Port=10
  HLSDem_KpNegLoCurr_mp : Outport  Port=11
  HLSDem_PWinPosLoCurr_mp : Outport  Port=12
  HLSDem_PWinNegLoCurr_mp : Outport  Port=13
  HLSDem_KiLoCurr_mp : Outport  Port=14
  HLSDem_KiPosLoCurr_mp : Outport  Port=15
  HLSDem_KiNegLoCurr_mp : Outport  Port=16
  HLSDem_IWinPosLoCurr_mp : Outport  Port=17
  HLSDem_IWinNegLoCurr_mp : Outport  Port=18
  HLSDem_KpHiCurr_mp : Outport  Port=19
  HLSDem_KpPosHiCurr_mp : Outport  Port=20
  HLSDem_KpNegHiCurr_mp : Outport  Port=21
  HLSDem_PWinPosHiCurr_mp : Outport  Port=22
  HLSDem_PWinNegHiCurr_mp : Outport  Port=23
  HLSDem_KiHiCurr_mp : Outport  Port=24
  HLSDem_KiPosHiCurr_mp : Outport  Port=25
  HLSDem_KiNegHiCurr_mp : Outport  Port=26
  HLSDem_IWinPosHiCurr_mp : Outport  Port=27
  HLSDem_IWinNegHiCurr_mp : Outport  Port=28
  wires:
  Limitation of the speed gradient/2(HLSDem_dnDeclLim) -> HLSDem_dnDeclLim/1
  HLSDem_KiCorFac_mp/1 -> Parameter Set/2(HLSDem_KiCorFac_mp)
  Selection of  outer feedback factor/2(HLSDem_facFdbkLo) -> HLSDem_facFdbkLo/1
  Limitation of the speed gradient/1(HLSDem_dnAccLim) -> HLSDem_dnAccLim/1
  Selection of  outer feedback factor/1(HLSDem_facFdbkHi) -> HLSDem_facFdbkHi/1
  Selection of inner feedback factor/4(HLSDem_InrtVehCurr) -> HLSDem_InrtVehCurr/1
  Selection of inner feedback factor/3(HLSDem_tiFltTrqLosEstCurr) -> HLSDem_tiFltTrqLosEstCurr/1
  Selection of inner feedback factor/2(HLSDem_facFdbkTrqLosHi) -> HLSDem_facFdbkTrqLosHi/1
  PT_rGrip/1 -> Selection of  outer feedback factor/1(PT_rGrip), Selection of inner feedback factor/2(PT_rGrip), Parameter Set/4(PT_rGrip)
  Selection of inner feedback factor/1(HLSDem_facFdbkTrqLosLo) -> HLSDem_facFdbkTrqLosLo/1
  GlbDa_rTrqTot/1 -> Parameter Set/3(GlbDa_rTrqTot), Selection of inner feedback factor/1(GlbDa_rTrqTot)
  HLSDem_KpCorFac_mp/1 -> Parameter Set/1(HLSDem_KpCorFac_mp)
  Parameter Set/13(HLSDem_KpNegHiCurr_mp) -> HLSDem_KpNegHiCurr_mp/1
  Parameter Set/2(HLSDem_KpPosLoCurr_mp) -> HLSDem_KpPosLoCurr_mp/1
  Parameter Set/7(HLSDem_KiPosLoCurr_mp) -> HLSDem_KiPosLoCurr_mp/1
  Parameter Set/20(HLSDem_IWinNegHiCurr_mp) -> HLSDem_IWinNegHiCurr_mp/1
  Parameter Set/15(HLSDem_PWinNegHiCurr_mp) -> HLSDem_PWinNegHiCurr_mp/1
  Parameter Set/11(HLSDem_KpHiCurr_mp) -> HLSDem_KpHiCurr_mp/1
  Parameter Set/4(HLSDem_PWinPosLoCurr_mp) -> HLSDem_PWinPosLoCurr_mp/1
  Parameter Set/6(HLSDem_KiLoCurr_mp) -> HLSDem_KiLoCurr_mp/1
  Parameter Set/3(HLSDem_KpNegLoCurr_mp) -> HLSDem_KpNegLoCurr_mp/1
  Parameter Set/8(HLSDem_KiNegLoCurr_mp) -> HLSDem_KiNegLoCurr_mp/1
  Parameter Set/5(HLSDem_PWinNegLoCurr_mp) -> HLSDem_PWinNegLoCurr_mp/1
  Parameter Set/9(HLSDem_IWinPosLoCurr_mp) -> HLSDem_IWinPosLoCurr_mp/1
  Parameter Set/17(HLSDem_KiPosHiCurr_mp) -> HLSDem_KiPosHiCurr_mp/1
  Parameter Set/19(HLSDem_IWinPosHiCurr_mp) -> HLSDem_IWinPosHiCurr_mp/1
  Parameter Set/10(HLSDem_IWinNegLoCurr_mp) -> HLSDem_IWinNegLoCurr_mp/1
  Parameter Set/1(HLSDem_KpLoCurr_mp) -> HLSDem_KpLoCurr_mp/1
  Parameter Set/12(HLSDem_KpPosHiCurr_mp) -> HLSDem_KpPosHiCurr_mp/1
  Parameter Set/14(HLSDem_PWinPosHiCurr_mp) -> HLSDem_PWinPosHiCurr_mp/1
  Parameter Set/16(HLSDem_KiHiCurr_mp) -> HLSDem_KiHiCurr_mp/1
  Parameter Set/18(HLSDem_KiNegHiCurr_mp) -> HLSDem_KiNegHiCurr_mp/1

== system HLSDem_SelectParameter/HLSDem_Parameter_Selection/Parameter_Correction/EngtFld_Selector ==
  TempSwt : Inport
  CEngDsT_t : Inport  Tag=deg  Description=engine coolant temperature after filter  Port=2
  Oil_tSwmp : Inport  Tag=deg  Description=Oil temperature in oil sump  Port=3
  EngDa_tEng : Inport  Tag=deg  Description=Engine temperature  Port=4
  Data Type Conversion : DataTypeConversion  OutDataTypeStr=uint8
  Multiport Switch : MultiPortSwitch  DataPortOrder=Zero-based contiguous
  EngDa_tFld_mp : Outport  Tag=deg  Description=Engine temperature field
  wires:
  CEngDsT_t/1 -> Multiport Switch/2
  Multiport Switch/1 -> EngDa_tFld_mp/1
  EngDa_tEng/1 -> Multiport Switch/4
  Oil_tSwmp/1 -> Multiport Switch/3
  Data Type Conversion/1 -> Multiport Switch/1
  TempSwt/1 -> Data Type Conversion/1

== system HLSDem_SelectParameter/HLSDem_Parameter_Selection/Parameter_Selection/Limitation of the speed gradient ==
  note: %configured=0%
  note: %减速梯度限值%
  note: %加速梯度限值%
  note: %正常情况下减速%
  note: %踩刹车减速%
  Constant1 : Constant  Value=HLSDem_NoGripdnAccLim_C
  Constant2 : Constant  Value=HLSDem_NoGripdnDeclLimBrk_C
  Constant4 : Constant  Value=0  OutDataTypeStr=Inherit: Inherit via back propagation
  Constant5 : Constant  Value=HLSDem_NoGripdnDeclLim_C
  Constant6 : Constant  Value=HLSDem_stBrkTrq_C
  Relational Operator1 : RelationalOperator  Operator=>  OutDataTypeStr=boolean  RndMeth=Nearest  InputSameDT=on
  Signal Conversion : SignalConversion  OverrideOpt=off
  Switch3 : Switch  Criteria=u2 ~= 0  InputSameDT=on
  HLSDem_dnAccLim : Outport
  HLSDem_dnDeclLim : Outport  Port=2
  wires:
  Constant4/1 -> Relational Operator1/2
  Constant6/1 -> Relational Operator1/1
  Constant2/1 -> Switch3/1
  Relational Operator1/1 -> Switch3/2
  Constant5/1 -> Switch3/3
  Switch3/1 -> HLSDem_dnDeclLim/1
  Constant1/1 -> Signal Conversion/1
  Signal Conversion/1 -> HLSDem_dnAccLim/1

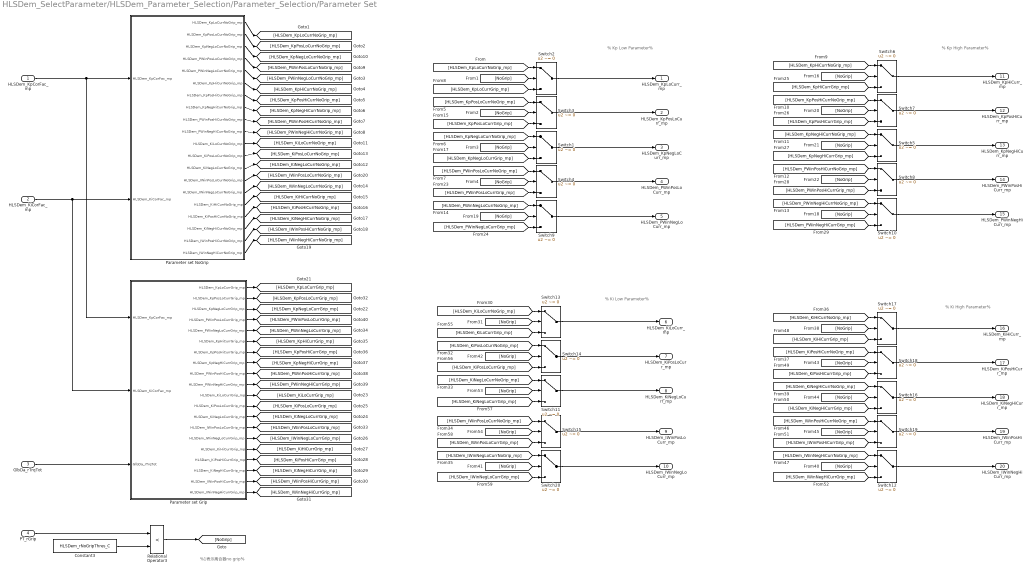
== system HLSDem_SelectParameter/HLSDem_Parameter_Selection/Parameter_Selection/Parameter Set ==
  note: %1表示离合器no grip%
  note: % Ki High Parameter%
  note: % Ki Low Parameter%
  note: % Kp High Parameter%
  note: % Kp Low Parameter%
  HLSDem_KpCorFac_mp : Inport
  HLSDem_KiCorFac_mp : Inport  Port=2
  GlbDa_rTrqTot : Inport  Port=3
  PT_rGrip : Inport  Port=4
  Constant3 : Constant  Value=HLSDem_rNoGripThres_C
  Parameter set Grip : Subsystem
  "Parameter set NoGrip " : Subsystem
  Relational Operator3 : RelationalOperator  Operator=<  OutDataTypeStr=boolean  RndMeth=Nearest
  Switch{1,3..20} (19 alike) : Switch  Criteria=u2 ~= 0
  Switch2 : Switch  Criteria=u2 ~= 0  InputSameDT=on
  HLSDem_KpLoCurr_mp : Outport
  HLSDem_KpPosLoCurr_mp : Outport  Port=2
  HLSDem_KpNegLoCurr_mp : Outport  Port=3
  HLSDem_PWinPosLoCurr_mp : Outport  Port=4
  HLSDem_PWinNegLoCurr_mp : Outport  Port=5
  HLSDem_KiLoCurr_mp : Outport  Port=6
  HLSDem_KiPosLoCurr_mp : Outport  Port=7
  HLSDem_KiNegLoCurr_mp : Outport  Port=8
  HLSDem_IWinPosLoCurr_mp : Outport  Port=9
  HLSDem_IWinNegLoCurr_mp : Outport  Port=10
  HLSDem_KpHiCurr_mp : Outport  Port=11
  HLSDem_KpPosHiCurr_mp : Outport  Port=12
  HLSDem_KpNegHiCurr_mp : Outport  Port=13
  HLSDem_PWinPosHiCurr_mp : Outport  Port=14
  HLSDem_PWinNegHiCurr_mp : Outport  Port=15
  HLSDem_KiHiCurr_mp : Outport  Port=16
  HLSDem_KiPosHiCurr_mp : Outport  Port=17
  HLSDem_KiNegHiCurr_mp : Outport  Port=18
  HLSDem_IWinPosHiCurr_mp : Outport  Port=19
  HLSDem_IWinNegHiCurr_mp : Outport  Port=20
  wires:
  Parameter set Grip/5(HLSDem_PWinNegLoCurrGrip_mp) -> [HLSDem_PWinNegLoCurrGrip_mp]
  Constant3/1 -> Relational Operator3/2
  "Parameter set NoGrip "/3(HLSDem_KpNegLoCurrNoGrip_mp) -> [HLSDem_KpNegLoCurrNoGrip_mp]
  Parameter set Grip/12(HLSDem_KiPosLoCurrGrip_mp) -> [HLSDem_KiPosLoCurrGrip_mp]
  "Parameter set NoGrip "/10(HLSDem_PWinNegHiCurrNoGrip_mp) -> [HLSDem_PWinNegHiCurrNoGrip_mp]
  Parameter set Grip/3(HLSDem_KpNegLoCurrGrip_mp) -> [HLSDem_KpNegLoCurrGrip_mp]
  Parameter set Grip/7(HLSDem_KpPosHiCurrGrip_mp) -> [HLSDem_KpPosHiCurrGrip_mp]
  "Parameter set NoGrip "/12(HLSDem_KiPosLoCurrNoGrip_mp) -> [HLSDem_KiPosLoCurrNoGrip_mp]
  "Parameter set NoGrip "/16(HLSDem_KiHiCurrNoGrip_mp) -> [HLSDem_KiHiCurrNoGrip_mp]
  "Parameter set NoGrip "/14(HLSDem_IWinPosLoCurrNoGrip_mp) -> [HLSDem_IWinPosLoCurrNoGrip_mp]
  Parameter set Grip/15(HLSDem_IWinNegLoCurrGrip_mp) -> [HLSDem_IWinNegLoCurrGrip_mp]
  Parameter set Grip/19(HLSDem_IWinPosHiCurrGrip_mp) -> [HLSDem_IWinPosHiCurrGrip_mp]
  "Parameter set NoGrip "/2(HLSDem_KpPosLoCurrNoGrip_mp) -> [HLSDem_KpPosLoCurrNoGrip_mp]
  HLSDem_KiCorFac_mp/1 -> Parameter set Grip/2(HLSDem_KiCorFac_mp), "Parameter set NoGrip "/2(HLSDem_KiCorFac_mp)
  Parameter set Grip/11(HLSDem_KiLoCurrGrip_mp) -> [HLSDem_KiLoCurrGrip_mp]
  Parameter set Grip/6(HLSDem_KpHiCurrGrip_mp) -> [HLSDem_KpHiCurrGrip_mp]
  "Parameter set NoGrip "/8(HLSDem_KpNegHiCurrNoGrip_mp) -> [HLSDem_KpNegHiCurrNoGrip_mp]
  HLSDem_KpCorFac_mp/1 -> Parameter set Grip/1(HLSDem_KpCorFac_mp), "Parameter set NoGrip "/1(HLSDem_KpCorFac_mp)
  Parameter set Grip/20(HLSDem_IWinNegHiCurrGrip_mp) -> [HLSDem_IWinNegHiCurrGrip_mp]
  "Parameter set NoGrip "/13(HLSDem_KiNegLoCurrNoGrip_mp) -> [HLSDem_KiNegLoCurrNoGrip_mp]
  Relational Operator3/1 -> [NoGrip]
  PT_rGrip/1 -> Relational Operator3/1
  Parameter set Grip/17(HLSDem_KiPosHiCurrGrip_mp) -> [HLSDem_KiPosHiCurrGrip_mp]
  Parameter set Grip/18(HLSDem_KiNegHiCurrGrip_mp) -> [HLSDem_KiNegHiCurrGrip_mp]
  GlbDa_rTrqTot/1 -> Parameter set Grip/3(GlbDa_rTrqTot)
  "Parameter set NoGrip "/15(HLSDem_IWinNegLoCurrNoGrip_mp) -> [HLSDem_IWinNegLoCurrNoGrip_mp]
  "Parameter set NoGrip "/19(HLSDem_IWinPosHiCurrNoGrip_mp) -> [HLSDem_IWinPosHiCurrNoGrip_mp]
  "Parameter set NoGrip "/20(HLSDem_IWinNegHiCurrNoGrip_mp) -> [HLSDem_IWinNegHiCurrNoGrip_mp]
  "Parameter set NoGrip "/1(HLSDem_KpLoCurrNoGrip_mp) -> [HLSDem_KpLoCurrNoGrip_mp]
  Parameter set Grip/1(HLSDem_KpLoCurrGrip_mp) -> [HLSDem_KpLoCurrGrip_mp]
  Parameter set Grip/14(HLSDem_IWinPosLoCurrGrip_mp) -> [HLSDem_IWinPosLoCurrGrip_mp]
  Parameter set Grip/16(HLSDem_KiHiCurrGrip_mp) -> [HLSDem_KiHiCurrGrip_mp]
  Parameter set Grip/9(HLSDem_PWinPosHiCurrGrip_mp) -> [HLSDem_PWinPosHiCurrGrip_mp]
  Parameter set Grip/13(HLSDem_KiNegLoCurrGrip_mp) -> [HLSDem_KiNegLoCurrGrip_mp]
  "Parameter set NoGrip "/4(HLSDem_PWinPosLoCurrNoGrip_mp) -> [HLSDem_PWinPosLoCurrNoGrip_mp]
  Parameter set Grip/4(HLSDem_PWinPosLoCurrGrip_mp) -> [HLSDem_PWinPosLoCurrGrip_mp]
  Parameter set Grip/2(HLSDem_KpPosLoCurrGrip_mp) -> [HLSDem_KpPosLoCurrGrip_mp]
  "Parameter set NoGrip "/17(HLSDem_KiPosHiCurrNoGrip_mp) -> [HLSDem_KiPosHiCurrNoGrip_mp]
  "Parameter set NoGrip "/6(HLSDem_KpHiCurrNoGrip_mp) -> [HLSDem_KpHiCurrNoGrip_mp]
  Parameter set Grip/10(HLSDem_PWinNegHiCurrGrip_mp) -> [HLSDem_PWinNegHiCurrGrip_mp]
  "Parameter set NoGrip "/5(HLSDem_PWinNegLoCurrNoGrip_mp) -> [HLSDem_PWinNegLoCurrNoGrip_mp]
  Parameter set Grip/8(HLSDem_KpNegHiCurrGrip_mp) -> [HLSDem_KpNegHiCurrGrip_mp]
  "Parameter set NoGrip "/7(HLSDem_KpPosHiCurrNoGrip_mp) -> [HLSDem_KpPosHiCurrNoGrip_mp]
  "Parameter set NoGrip "/18(HLSDem_KiNegHiCurrNoGrip_mp) -> [HLSDem_KiNegHiCurrNoGrip_mp]
  "Parameter set NoGrip "/11(HLSDem_KiLoCurrNoGrip_mp) -> [HLSDem_KiLoCurrNoGrip_mp]
  "Parameter set NoGrip "/9(HLSDem_PWinPosHiCurrNoGrip_mp) -> [HLSDem_PWinPosHiCurrNoGrip_mp]
  Switch18/1 -> HLSDem_KiPosHiCurr_mp/1
  Switch16/1 -> HLSDem_KiNegHiCurr_mp/1
  [NoGrip] -> Switch19/2
  Switch17/1 -> HLSDem_KiHiCurr_mp/1
  [NoGrip] -> Switch16/2
  [NoGrip] -> Switch12/2
  [HLSDem_KpLoCurrNoGrip_mp] -> Switch2/1
  Switch12/1 -> HLSDem_IWinNegHiCurr_mp/1
  [HLSDem_KiHiCurrNoGrip_mp] -> Switch17/1
  [HLSDem_KiNegLoCurrGrip_mp] -> Switch11/3
  [HLSDem_KiPosHiCurrNoGrip_mp] -> Switch18/1
  [HLSDem_IWinPosHiCurrNoGrip_mp] -> Switch19/1
  [HLSDem_KiNegHiCurrNoGrip_mp] -> Switch16/1
  [HLSDem_KiPosLoCurrGrip_mp] -> Switch14/3
  [HLSDem_KiLoCurrGrip_mp] -> Switch13/3
  Switch19/1 -> HLSDem_IWinPosHiCurr_mp/1
  [NoGrip] -> Switch18/2
  [HLSDem_IWinPosHiCurrGrip_mp] -> Switch19/3
  [HLSDem_IWinNegHiCurrGrip_mp] -> Switch12/3
  [HLSDem_KiPosHiCurrGrip_mp] -> Switch18/3
  [HLSDem_KiNegHiCurrGrip_mp] -> Switch16/3
  [HLSDem_KiHiCurrGrip_mp] -> Switch17/3
  [HLSDem_KiPosLoCurrNoGrip_mp] -> Switch14/1
  [HLSDem_IWinNegHiCurrNoGrip_mp] -> Switch12/1
  [HLSDem_KiLoCurrNoGrip_mp] -> Switch13/1
  [HLSDem_IWinPosLoCurrNoGrip_mp] -> Switch15/1
  [HLSDem_PWinNegLoCurrGrip_mp] -> Switch9/3
  [HLSDem_KpHiCurrGrip_mp] -> Switch6/3
  [HLSDem_KpPosLoCurrGrip_mp] -> Switch3/3
  [HLSDem_KpNegLoCurrGrip_mp] -> Switch1/3
  [HLSDem_PWinPosLoCurrGrip_mp] -> Switch4/3
  [HLSDem_KpPosHiCurrGrip_mp] -> Switch7/3
  [HLSDem_KpNegHiCurrNoGrip_mp] -> Switch5/1
  [NoGrip] -> Switch15/2
  [HLSDem_PWinNegHiCurrGrip_mp] -> Switch10/3
  Switch15/1 -> HLSDem_IWinPosLoCurr_mp/1
  [NoGrip] -> Switch13/2
  [NoGrip] -> Switch11/2
  [NoGrip] -> Switch14/2
  [HLSDem_KpNegLoCurrNoGrip_mp] -> Switch1/1
  [HLSDem_PWinPosLoCurrNoGrip_mp] -> Switch4/1
  Switch13/1 -> HLSDem_KiLoCurr_mp/1
  [HLSDem_KiNegLoCurrNoGrip_mp] -> Switch11/1
  [NoGrip] -> Switch17/2
  Switch14/1 -> HLSDem_KiPosLoCurr_mp/1
  [HLSDem_IWinNegLoCurrNoGrip_mp] -> Switch20/1
  Switch11/1 -> HLSDem_KiNegLoCurr_mp/1
  Switch20/1 -> HLSDem_IWinNegLoCurr_mp/1
  [NoGrip] -> Switch20/2
  [HLSDem_KpNegHiCurrGrip_mp] -> Switch5/3
  [HLSDem_PWinPosHiCurrGrip_mp] -> Switch8/3
  [HLSDem_PWinPosHiCurrNoGrip_mp] -> Switch8/1
  [HLSDem_KpLoCurrGrip_mp] -> Switch2/3
  [HLSDem_KpHiCurrNoGrip_mp] -> Switch6/1
  Switch6/1 -> HLSDem_KpHiCurr_mp/1
  Switch5/1 -> HLSDem_KpNegHiCurr_mp/1
  [NoGrip] -> Switch10/2
  Switch10/1 -> HLSDem_PWinNegHiCurr_mp/1
  Switch7/1 -> HLSDem_KpPosHiCurr_mp/1
  [NoGrip] -> Switch8/2
  Switch9/1 -> HLSDem_PWinNegLoCurr_mp/1
  Switch8/1 -> HLSDem_PWinPosHiCurr_mp/1
  [NoGrip] -> Switch6/2
  [NoGrip] -> Switch5/2
  [NoGrip] -> Switch7/2
  [HLSDem_IWinPosLoCurrGrip_mp] -> Switch15/3
  [HLSDem_IWinNegLoCurrGrip_mp] -> Switch20/3
  [NoGrip] -> Switch4/2
  [NoGrip] -> Switch1/2
  Switch2/1 -> HLSDem_KpLoCurr_mp/1
  [NoGrip] -> Switch3/2
  Switch4/1 -> HLSDem_PWinPosLoCurr_mp/1
  [NoGrip] -> Switch2/2
  Switch1/1 -> HLSDem_KpNegLoCurr_mp/1
  Switch3/1 -> HLSDem_KpPosLoCurr_mp/1
  [HLSDem_KpPosHiCurrNoGrip_mp] -> Switch7/1
  [HLSDem_PWinNegHiCurrNoGrip_mp] -> Switch10/1
  [HLSDem_PWinNegLoCurrNoGrip_mp] -> Switch9/1
  [NoGrip] -> Switch9/2
  [HLSDem_KpPosLoCurrNoGrip_mp] -> Switch3/1

== system HLSDem_SelectParameter/HLSDem_Parameter_Selection/Parameter_Selection/Selection of  outer feedback factor ==
  PT_rGrip : Inport
  Constant1 : Constant  Value=0  OutDataTypeStr=Inherit: Inherit via back propagation
  Constant2 : Constant  Value=HLSDem_facFdbkLoGrip_C
  Constant3 : Constant  Value=HLSDem_facFdbkLoNoGrip_C
  Constant4 : Constant  Value=HLSDem_rNoGripThres_C
  Data Type Conversion : DataTypeConversion
  Logical Operator2 : Logic  Operator=NOT  AllPortsSameDT=off  OutDataTypeStr=boolean
  Relational Operator1 : RelationalOperator  Operator=<  OutDataTypeStr=boolean  RndMeth=Nearest  InputSameDT=on
  Switch5 : Switch  Criteria=u2 ~= 0  InputSameDT=on
  HLSDem_facFdbkHi : Outport
  HLSDem_facFdbkLo : Outport  Port=2
  wires:
  Constant4/1 -> Relational Operator1/2
  Constant3/1 -> Switch5/3
  Logical Operator2/1 -> Switch5/2
  Constant1/1 -> Data Type Conversion/1
  PT_rGrip/1 -> Relational Operator1/1
  Relational Operator1/1 -> Logical Operator2/1
  Constant2/1 -> Switch5/1
  Switch5/1 -> HLSDem_facFdbkLo/1
  Data Type Conversion/1 -> HLSDem_facFdbkHi/1
